simulink model "test_pow_sim_1_loop"  (R2015a)
settings: Solver=FixedStepDiscrete  StartTime=0.0  StopTime=0.5  FixedStep=1  RelTol=1e-3
libraries: dspsrcs4 x2, powerlib x1
settings Model: Creator=metr  LastModifiedBy=metr

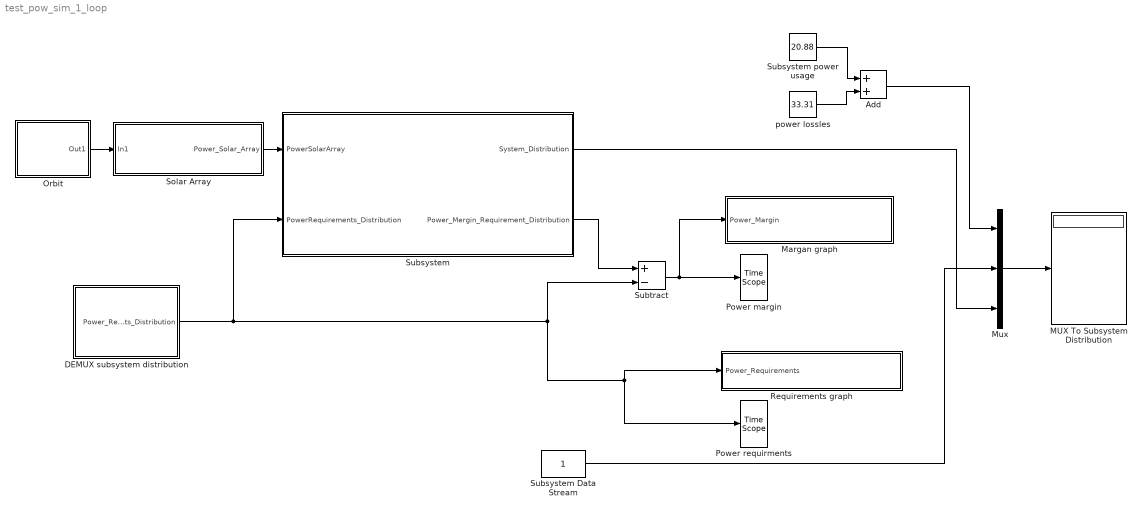
== system test_pow_sim_1_loop ==
  Add : Sum
  DEMUX subsystem distribution : Subsystem
  MUX To Subsystem Distribution : Display
  Margan graph : MATLAB Function  TreatAsAtomicUnit=on
  Mux : Mux  Inputs=3
  Orbit : Subsystem
  "Power margin " : TimeScope
  Power requirments : TimeScope
  Requirements graph : MATLAB Function  TreatAsAtomicUnit=on
  Solar Array : Subsystem
  Subsystem : Subsystem
  Subsystem Data Stream : Constant
  Subsystem power usage : Constant  Value=20.88
  Subtract : Sum  Inputs=+-
  power lossles : Constant  Value=33.31
  wires:
  Mux/1 -> MUX To Subsystem Distribution/1
  Add/1 -> Mux/1
  Subsystem power usage/1 -> Add/1
  power lossles/1 -> Add/2
  Subsystem Data Stream/1 -> Mux/2
  Subtract/1 -> "Power margin "/1, Margan graph/1(Power_Margin)
  DEMUX subsystem distribution/1(Power_Requirements_Distribution) -> Power requirments/1, Requirements graph/1(Power_Requirements), Subtract/2, Subsystem/2(PowerRequirements_Distribution)
  Subsystem/1(System_Distribution) -> Mux/3
  Subsystem/2(Power_Mergin_Requirement_Distribution) -> Subtract/1
  Orbit/1(Out1) -> Solar Array/1(In1)
  Solar Array/1(Power_Solar_Array) -> Subsystem/1(PowerSolarArray)

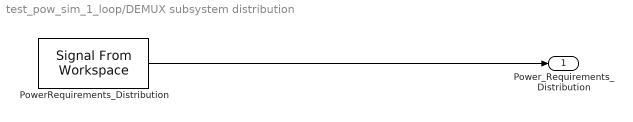
== system test_pow_sim_1_loop/DEMUX subsystem distribution ==
  PowerRequirements_Distribution : dspsrcs4/Signal From Workspace  X="[3.5          3.5          3.5          3.5          3.5          3.5          3.5          3.5          3.5          3.5          3.5          3.5          3.5          3.5          3.5          3.5          3.5          3.5          3.5          3.5          3.5          3.5          3.5          3.5          3.5          3.5          3.5          3.5          3.5          3.5          3.5          3.5          3.5          3.5          3.5          3.5          3.5          3.5          3.5          3.5          3.5          3.5          3.5          3.5          3.5          3.5          3.5          3.5          3.5          3.5          3.5          3.5          3.5          3.5          3.5          3.5          3.5          3.5          3.5          3.5          3.5          3.5          3.5          3.5          3.5          3.5          3.5          3.5          3.5          3.5          3.5          3.5          3.5          3.5          3.5          3.5          3.5          3.5          3.5          3.5         10.5         10.5         10.5         10.5         10.5         10.5         10.5         10.5         10.5         10.5          3.5          3.5          3.5          3.5          3.5          3.5          3.5          3.5          3.5          3.5          3.5          3.5          3.5          3.5          3.5          3.5          3.5          3.5          3.5          3.5          3.5          3.5          3.5          3.5          3.5          3.5          3.5          3.5          3.5          3.5          3.5          3.5          3.5          3.5          3.5          3.5          3.5          3.5          3.5          3.5          3.5          3.5          3.5          3.5          3.5          3.5          3.5          3.5          3.5          3.5          3.5          3.5          3.5          3.5          3.5          3.5          3.5          3.5          3.5          3.5          3.5          3.5          3.5          3.5          3.5          3.5          3.5          3.5          3.5          3.5          3.5          3.5          3.5          3.5          3.5          3.5          3.5          3.5          3.5          3.5         10.5         10.5         10.5         10.5         10.5         10.5         10.5         10.5         10.5         10.5          3.5          3.5          3.5          3.5          3.5          3.5          3.5          3.5          3.5          3.5          3.5          3.5          3.5          3.5          3.5          3.5          3.5          3.5          3.5          3.5          3.5          3.5          3.5          3.5          3.5          3.5          3.5          3.5          3.5          3.5          3.5          3.5          3.5          3.5          3.5          3.5          3.5          3.5          3.5          3.5          3.5          3.5          3.5          3.5          3.5          3.5          3.5          3.5          3.5          3.5          3.5          3.5          3.5          3.5          3.5          3.5          3.5          3.5          3.5          3.5          3.5          3.5          3.5          3.5          3.5          3.5          3.5          3.5          3.5          3.5          3.5          3.5          3.5          3.5          3.5          3.5          3.5          3.5          3.5          3.5         10.5         10.5         10.5         10.5         10.5         10.5         10.5         10.5         10.5         10.5          3.5          3.5          3.5          3.5          3.5          3.5          3.5          3.5          3.5          3.5          3.5          3.5          3.5          3.5          3.5          3.5          3.5          3.5          3.5          3.5          3.5          3.5          3.5          3.5          3.5          3.5          3.5          3.5          3.5          3.5          3.5          3.5          3.5          3.5          3.5          3.5          3.5          3.5 ...(+14712 chars)]"  Ts=689  nsamps=689  OutputAfterFinalValue=Cyclic repetition  ignoreOrWarnInputAndFrameLengths=on
  Power_Requirements_Distribution : Outport
  wires:
  PowerRequirements_Distribution/1 -> Power_Requirements_Distribution/1

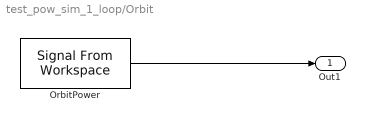
== system test_pow_sim_1_loop/Orbit ==
  OrbitPower : dspsrcs4/Signal From Workspace  X="[0      1.0629      1.1204      1.1735      1.2218      1.2652      1.3035      1.3364      1.3639      1.3857      1.4016      1.4117      1.4157      1.4137      1.4056      1.3916      1.3718      1.3463      1.3154      1.2795      1.2389      1.1941      1.1455      1.0935      1.0387      1.0216      1.0753      1.1245      1.1692      1.2095      1.2456      1.2777      1.3058      1.3303      1.3513       1.369      1.3835      1.3952      1.4041      1.4104      1.4144       1.416           0           0           0           0           0           0           0           0           0           0           0           0           0           0           0           0           0           0           0           0           0           0           0           0           0           0           0           0           0           0           0           0           0           0           0           0           0           0           0           0           0           0           0           0           0           0           0           0       1.416      1.4129      1.4074      1.3991      1.3878      1.3735      1.3557      1.3344      1.3094      1.2803       1.247      1.2092      1.1669      1.1198      1.0679      1.0111      1.0532      1.1094      1.1624      1.2115      1.2563      1.2963       1.331      1.3602      1.3835      1.4008      1.4119      1.4168      1.4154      1.4079      1.3943      1.3749      1.3498      1.3192      1.2833      1.2425      1.1968      1.1467      1.0922      1.0336      1.0337       1.092       1.146      1.1955      1.2404      1.2805      1.3157      1.3459      1.3709      1.3906       1.405      1.4139      1.4173      1.4151      1.4075      1.3945      1.3761      1.3527      1.3243      1.2912      1.2537      1.2122      1.1671      1.1187      1.0673      1.0135      1.0469      1.0969      1.1427      1.1845      1.2224      1.2563      1.2866      1.3133      1.3365      1.3565      1.3733      1.3872      1.3983      1.4068      1.4127      1.4163      1.4176           0           0           0           0           0           0           0           0           0           0           0           0           0           0           0           0           0           0           0           0           0           0           0           0           0           0           0           0           0           0           0           0           0           0           0           0           0           0           0           0           0           0           0           0           0           0      1.4147      1.4088      1.3998      1.3874      1.3714      1.3515      1.3276      1.2994      1.2667      1.2292      1.1869      1.1396      1.0872      1.0298      1.0396      1.0983      1.1534      1.2044      1.2507      1.2919      1.3277      1.3578      1.3819         1.4       1.412      1.4178      1.4177      1.4116      1.3999      1.3828      1.3603      1.3329      1.3007       1.264       1.223      1.1779      1.1291      1.0766      1.0208      1.0454      1.0992      1.1491      1.1952      1.2372       1.275      1.3086       1.338      1.3629      1.3833      1.3992      1.4104      1.4169      1.4188      1.4158      1.4082      1.3958      1.3788      1.3573      1.3313      1.3011      1.2668      1.2288      1.1871      1.1422      1.0942      1.0436      1.0187      1.0695      1.1166      1.1601      1.1998       1.236      1.2685      1.2976      1.3232      1.3455      1.3646      1.3806      1.3937      1.4039      1.4115      1.4164      1.4188           0           0           0           0           0           0           0           0           0           0           0           0           0           0           0           0           0           0           0           0           0           0           0           0           0           0           0           0           0           0           0           0 ...(+4259 chars)]"  Ts=689  nsamps=689  OutputAfterFinalValue=Setting to zero  ignoreOrWarnInputAndFrameLengths=off
  Out1 : Outport
  wires:
  OrbitPower/1 -> Out1/1

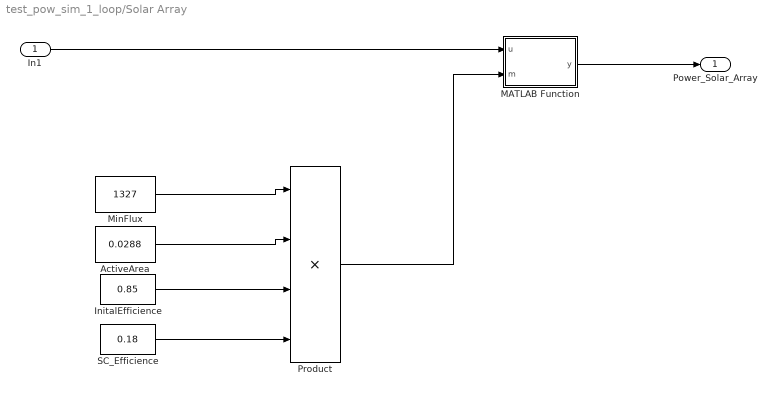
== system test_pow_sim_1_loop/Solar Array ==
  In1 : Inport
  ActiveArea : Constant  Value=0.0288
  InitalEfficience : Constant  Value=0.85
  MATLAB Function : MATLAB Function  TreatAsAtomicUnit=on
  MinFlux : Constant  Value=1327
  Product : Product  Inputs=4
  SC_Efficience : Constant  Value=0.18
  Power_Solar_Array : Outport
  wires:
  MinFlux/1 -> Product/1
  ActiveArea/1 -> Product/2
  InitalEfficience/1 -> Product/3
  SC_Efficience/1 -> Product/4
  MATLAB Function/1(y) -> Power_Solar_Array/1
  In1/1 -> MATLAB Function/1(u)
  Product/1 -> MATLAB Function/2(m)

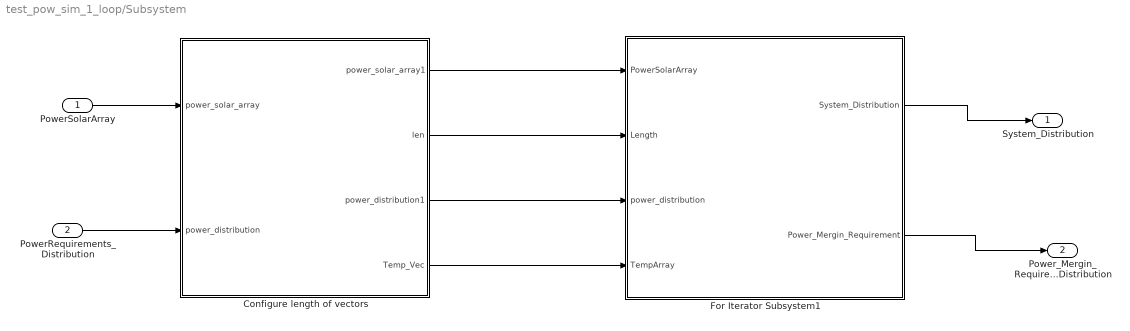
== system test_pow_sim_1_loop/Subsystem ==
  PowerSolarArray : Inport
  PowerRequirements_Distribution : Inport  Port=2
  Configure length of vectors : MATLAB Function  TreatAsAtomicUnit=on
  For Iterator Subsystem1 : Subsystem  TreatAsAtomicUnit=on
  System_Distribution : Outport
  Power_Mergin_Requirement_Distribution : Outport  Port=2
  wires:
  PowerRequirements_Distribution/1 -> Configure length of vectors/2(power_distribution)
  PowerSolarArray/1 -> Configure length of vectors/1(power_solar_array)
  Configure length of vectors/2(len) -> For Iterator Subsystem1/2(Length)
  For Iterator Subsystem1/1(System_Distribution) -> System_Distribution/1
  Configure length of vectors/1(power_solar_array1) -> For Iterator Subsystem1/1(PowerSolarArray)
  For Iterator Subsystem1/2(Power_Mergin_Requirement) -> Power_Mergin_Requirement_Distribution/1
  Configure length of vectors/3(power_distribution1) -> For Iterator Subsystem1/3(power_distribution)
  Configure length of vectors/4(Temp_Vec) -> For Iterator Subsystem1/4(TempArray)

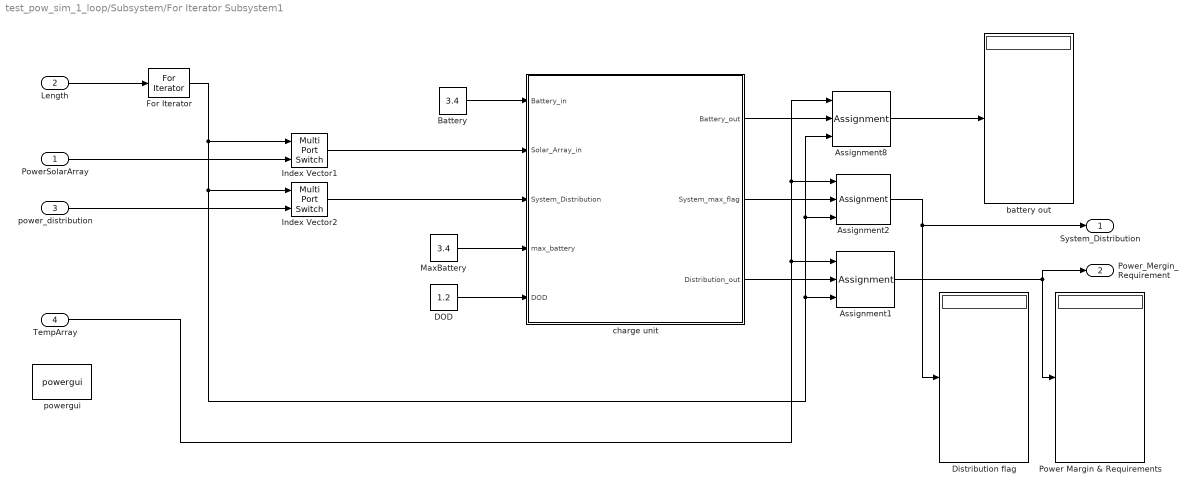
== system test_pow_sim_1_loop/Subsystem/For Iterator Subsystem1 ==
  PowerSolarArray : Inport
  Length : Inport  Port=2
  power_distribution : Inport  Port=3
  TempArray : Inport  Port=4
  Assignment1 : Assignment  DiagnosticForDimensions=Warning  IndexOptions=Index vector (port)
  Assignment2 : Assignment  DiagnosticForDimensions=Warning  IndexOptions=Index vector (port)
  Assignment8 : Assignment  DiagnosticForDimensions=Warning  IndexOptions=Index vector (port)
  Battery : Constant  Value=3.4
  DOD : Constant  Value=1.2
  Distribution flag : Display
  For Iterator : ForIterator  IterationSource=external  IterationLimit=1  IterationVariableDataType=double
  Index Vector1 : MultiPortSwitch  Inputs=1  DataPortIndices={2,3}
  Index Vector2 : MultiPortSwitch  Inputs=1  DataPortIndices={2,3}
  MaxBattery : Constant  Value=3.4
  Power Margin & Requirements : Display
  battery out : Display
  "charge unit " : MATLAB Function  TreatAsAtomicUnit=on
  powergui : powerlib/powergui  Priority=1  SimulationMode=Discrete  SolverType=Tustin/Backward Euler (TBE)  SampleTime=1  frequency=60  SPID=off  DisableSnubberDevices=off  DisableRonSwitches=off  DisableVfSwitches=off  SwTol=0  DisplayEquations=off  Interpol=off  methode=off  Ts=100  FunctionMessages=off  echomessages=off  HookPort=off  EnableUseOfTLC=off  x0status=blocks  frequencyindice=0  Pbase=100e6  ErrMax=1e-4  Iterations=1  UnitsV=kV  UnitsW=MW  buscounter=0  RestoreLinks=warning  ResistiveCurrentMeasurement=off  Frange=[0:2:500]  Ylog=off  Xlog=on  ShowGrid=off  save=off  variable=ZData  structure=0  ZoomFFT=off  StartTime=0.0  cycles=1  DisplayStyle=1  fundamental=60  FreqAxis=off  MaxFrequency=1000  frequencyindicesteady=1  RmsSteady=1  display=off
  System_Distribution : Outport
  Power_Mergin_Requirement : Outport  Port=2
  wires:
  PowerSolarArray/1 -> Index Vector1/2
  Length/1 -> For Iterator/1
  power_distribution/1 -> Index Vector2/2
  MaxBattery/1 -> "charge unit "/4(max_battery)
  Assignment2/1 -> System_Distribution/1, Distribution flag/1
  "charge unit "/1(Battery_out) -> Assignment8/2
  "charge unit "/3(Distribution_out) -> Assignment1/2
  "charge unit "/2(System_max_flag) -> Assignment2/2
  For Iterator/1 -> Index Vector1/1, Assignment8/3, Assignment2/3, Assignment1/3, Index Vector2/1
  DOD/1 -> "charge unit "/5(DOD)
  Battery/1 -> "charge unit "/1(Battery_in)
  TempArray/1 -> Assignment8/1, Assignment2/1, Assignment1/1
  Index Vector2/1 -> "charge unit "/3(System_Distribution)
  Index Vector1/1 -> "charge unit "/2(Solar_Array_in)
  Assignment8/1 -> battery out/1
  Assignment1/1 -> Power_Mergin_Requirement/1, Power Margin & Requirements/1

== matlab function test_pow_sim_1_loop/Solar Array/MATLAB Function ==
  data: u input; y output; m input
function y = fcn(u,m)
%#codegen
% u(1:10)
% m
y = u*m;
% y(1:10)
% hh=y(1:10)-3.5
% 'finished mutiply'

Total_Power_Generated=y;
coder.extrinsic('legend')
figure;
time=(1:length(Total_Power_Generated));
plot(time ,Total_Power_Generated),grid on
xlabel('time (seconds)');
ylabel( 'Total Power Generated(Wat)');
legend('Total Power Generated');
title('Total Power Generated');
xlim([0 max(time)])

== matlab function test_pow_sim_1_loop/Subsystem/Configure length of vectors ==
  data: power_solar_array1 output; len output; power_solar_array input; power_distribution input; power_distribution1 output; Temp_Vec output
function [power_solar_array1,len,power_distribution1,Temp_Vec] = fcn(power_solar_array,power_distribution)


power_solar_array1=power_solar_array;
len=length(power_solar_array);
power_distribution1 = power_distribution(mod(0:len-1, numel(power_distribution)) + 1);
Temp_Vec=zeros(len,1);

== matlab function test_pow_sim_1_loop/Margan graph ==
  data: Power_Margin input
function  GraphMargin( Power_Margin)
coder.extrinsic('legend')
coder.extrinsic('exist')
coder.extrinsic('delete')


figure;
time=(1:length(Power_Margin))
plot(time ,Power_Margin),grid on
xlabel('time (seconds)');
ylabel( 'Power Margin(Wat)');
legend(' Power Margin');
title('Power Margin');
xlim([0 max(time)])
bbb=99999

x=[ time' , Power_Margin]
A=size(x)
B=size(Power_Margin)
filename = 'Power_Margin.xlsx'

if ~exist(filename,'file')
    delete(filename); 
end


sheet = 2;
xlRange = 'E1';
xlswrite(filename,Power_Margin)

y='p'

== matlab function test_pow_sim_1_loop/Requirements graph ==
  data: Power_Requirements input
function  Graph_Requirements(Power_Requirements)

figure;
coder.extrinsic('legend')
 time=(1:length(Power_Requirements));
plot(time ,Power_Requirements),grid on
    xlabel('time (seconds)');
    ylabel( 'Power Requirements(Wat)');
    legend(' Power Requirements');
    title('Power Requirements');
     xlim([0 max(time)])

== matlab function test_pow_sim_1_loop/Subsystem/For Iterator Subsystem1/charge unit  ==
  data: Battery_out output; System_max_flag output; Battery_in input; Distribution_out output; Solar_Array_in input; System_Distribution input; max_battery input; DOD input
function [Battery_out,System_max_flag,Distribution_out] = fcn(Battery_in,Solar_Array_in,System_Distribution,max_battery,DOD)
coder.extrinsic('get_param');
coder.extrinsic('set_param');
coder.extrinsic('num2str');
coder.extrinsic('str2num');

x = double(0);
x=str2num(get_param('test_pow_sim_1_loop/Subsystem/For Iterator Subsystem1/Battery','Value'));
Battery_in=x+0


power_waste=0;
System_max_flag=0;
if(Solar_Array_in>=(System_Distribution))
    'greater or equal';
    Distribution_out = System_Distribution;
    Solar_Array_in=Solar_Array_in-(System_Distribution);
    
    if(Solar_Array_in>0 && Battery_in < max_battery)
        
        Battery_out=Solar_Array_in+Battery_in;
        
        if(Battery_out>max_battery)
            Battery_out=max_battery;
            System_max_flag=1;
            Solar_Array_in = Solar_Array_in - (Battery_out - Battery_in);
            power_waste=Solar_Array_in;
        end
    else
        if(Battery_in >= max_battery)
            System_max_flag=1;
        end
        Battery_out=Battery_in;
        power_waste=Solar_Array_in
    end
else% what is the value of x,y,z here ?
    'less than'
    Distribution_out=0;
    Battery_out=Battery_in;
    %%%%%if we can store them in battery
    if(Solar_Array_in>0 && Battery_in < max_battery)
        
        Battery_out=Solar_Array_in+Battery_in;
        
        if(Battery_out>max_battery)
            Battery_out=max_battery;
            System_max_flag=1;
            Solar_Array_in = Solar_Array_in - (Battery_out - Battery_in);
            power_waste=Solar_Array_in;
        end
    else
        if(Battery_in >= max_battery)
        System_max_flag=1;
        end
       
        Battery_out=Battery_in;
        power_waste=Solar_Array_in;
    end
    
    if(Battery_out >= (System_Distribution) && DOD <=(Battery_out-(System_Distribution)))
        
       
        Distribution_out = System_Distribution;
        
        Battery_out=Battery_out-(System_Distribution);
        System_max_flag=0;
        
    end
    
end

Distribution_out=Distribution_out+power_waste
set_param('test_pow_sim_1_loop/Subsystem/For Iterator Subsystem1/Battery','Value',num2str(Battery_out));

end
